simulink model "DC_motor_model"  (R2023a)
settings: Solver=VariableStepAuto  StartTime=0.0  StopTime=10  FixedStep=1/20000  MaxStep=1/10000  RelTol=1e-3
undefined symbols (not defined in the file or in its folder): sigbuilder_block
settings Model: Creator=SC34573  LastModifiedBy=Test
settings SolverCC: ZeroCrossAlgorithm=Adaptive  AlgebraicLoopSolver=TrustRegion
settings DebuggingCC: IgnoredZcDiagnostic=none  UnconnectedInputMsg=warning  UnconnectedOutputMsg=warning  UnconnectedLineMsg=warning
settings ModelReferenceCC: EnableRefExpFcnMdlSchedulingChecks=on
settings RTWCC: DLArmComputeVersion=19.05

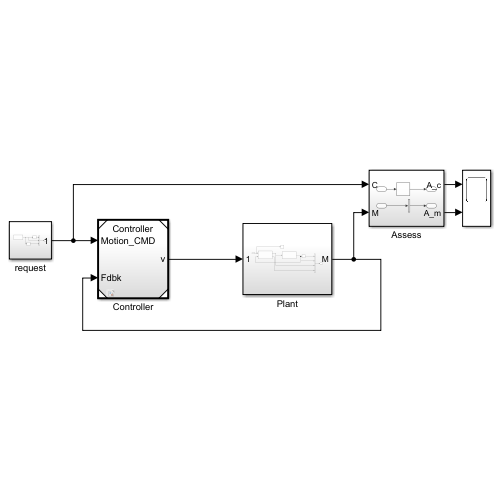
[thumbnail: Simulink's stored preview of the top-level diagram]
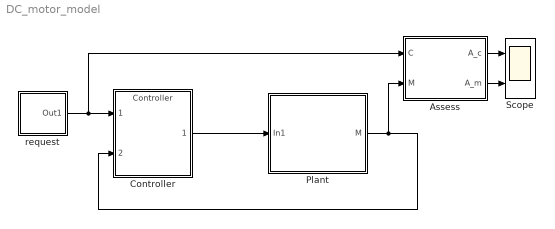
== system DC_motor_model ==
  Assess : Subsystem
  Controller : ModelReference  ModelNameDialog=Controller  SimulationMode=Normal  ModelReferenceVersion=1.31
  Plant : Subsystem
  Scope : Scope  NumInputPorts=2
  request : Subsystem
  wires:
  request/1(Out1) -> Assess/1(C), Controller/1
  Controller/1 -> Plant/1(In1)
  Plant/1(M) -> Controller/2, Assess/2(M)
  Assess/1(A_c) -> Scope/1
  Assess/2(A_m) -> Scope/2

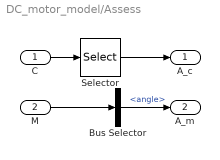
== system DC_motor_model/Assess ==
  C : Inport
  M : Inport  Port=2
  Bus Selector : BusSelector  OutputSignals=angle
  Selector : Selector  InputPortWidth=3  IndexOptions=Index vector (dialog)  Indices=1  OutputSizes=1
  A_c : Outport
  A_m : Outport  Port=2
  wires:
  Selector/1 -> A_c/1
  C/1 -> Selector/1
  M/1 -> Bus Selector/1
  Bus Selector/1 -> A_m/1  "<angle>"

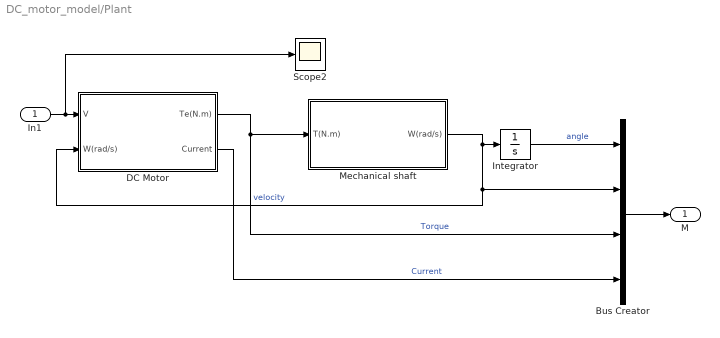
== system DC_motor_model/Plant ==
  In1 : Inport
  Bus Creator : BusCreator  Inputs=4
  "DC Motor " : Subsystem  mask{Vn=30, Tstall=20, wNL=20, L=1e-10}
      mask prompts: Vn "Nominal Voltage"; Tstall "Stall Torque(N.m)"; wNL "No Load Speed(rad/s)"; L "Inductance(H)"
      mask init:
      | K=Vn/wNL;
      | R=Vn^2/wNL/Tstall;
  Integrator : Integrator
  Mechanical shaft : Subsystem  mask{J=1, b=0}
      mask prompts: J "Shaft inertia(Kg.m^2)"; b "Damping Coefficient"
  Scope2 : Scope
  M : Outport
  wires:
  Mechanical shaft/1(W(rad/s)) -> "DC Motor "/2(W(rad/s)), Bus Creator/2, Integrator/1  "velocity"
  In1/1 -> Scope2/1, "DC Motor "/1(V)
  "DC Motor "/1(Te(N.m)) -> Bus Creator/3, Mechanical shaft/1(T(N.m))  "Torque"
  Integrator/1 -> Bus Creator/1  "angle"
  "DC Motor "/2(Current) -> Bus Creator/4  "Current"
  Bus Creator/1 -> M/1

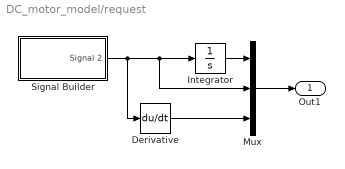
== system DC_motor_model/request ==
  Derivative : Derivative
  Integrator : Integrator
  Mux : Mux  Inputs=3
  Signal Builder : Subsystem  Tag=STV Subsys  LoadFcn=sigbuilder_block('load');  StartFcn=sigbuilder_block('start');  StopFcn=sigbuilder_block('stop');  ClipboardFcn=sigbuilder_block('clipboard');  mask(Sigbuilder block){tuvar=[0:10]}
      mask help: Simulink:masks:SigbuilderBlock_MD
      mask init:
      | if ~strcmp(get_param(bdroot(gcbh),'SimulationStatus'),'stopped') tuvar = sigbuilder_block('maskInit'); end
      settings: CopyFcn=sigbuilder_block('copy');  DeleteFcn=sigbuilder_block('delete');  ModelCloseFcn=sigbuilder_block('modelClose');  PreSaveFcn=sigbuilder_block('preSave');  PauseFcn=sigbuilder_block('pause');  ContinueFcn=sigbuilder_block('continue');  NameChangeFcn=sigbuilder_block('namechange');  OpenFcn=sigbuilder_block('open',[6 22.5 1420.5 635.25 ]);  CloseFcn=sigbuilder_block('close');
      mask Display: plot(0, 0, 100, 100,[2, 2, 32, 32, 2], [68, 8, 8, 68, 68],[32, 2], [38, 38], [32, 19, 2],[53, 60, 44], [32, 17, 17, 2],[16, 16, 31, 31]);txt = getActiveGroup(gcbh);text(2, 100, txt,'verticalAlignment', 'top');
  Out1 : Outport
  wires:
  Signal Builder/1(Signal 2) -> Mux/2, Integrator/1, Derivative/1
  Integrator/1 -> Mux/1
  Derivative/1 -> Mux/3
  Mux/1 -> Out1/1

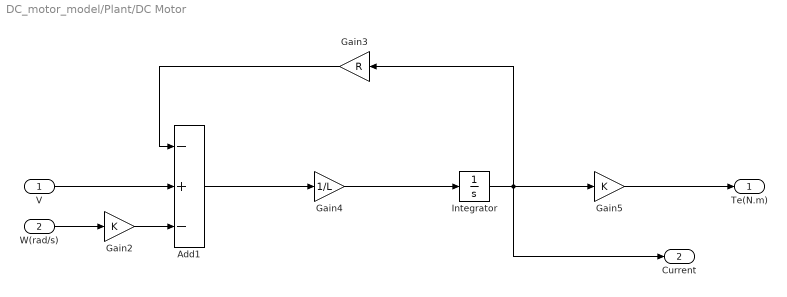
== system DC_motor_model/Plant/DC Motor  ==
  V : Inport
  W(rad/s) : Inport  Port=2
  Add1 : Sum  Inputs=-+-
  Gain2 : Gain  Gain=K
  Gain3 : Gain  Gain=R
  Gain4 : Gain  Gain=1/L
  Gain5 : Gain  Gain=K
  Integrator : Integrator
  Te(N.m) : Outport
  Current : Outport  Port=2
  wires:
  Integrator/1 -> Current/1, Gain5/1, Gain3/1
  V/1 -> Add1/2
  Add1/1 -> Gain4/1
  Gain4/1 -> Integrator/1
  W(rad/s)/1 -> Gain2/1
  Gain5/1 -> Te(N.m)/1
  Gain2/1 -> Add1/3
  Gain3/1 -> Add1/1

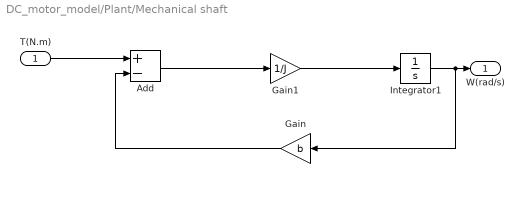
== system DC_motor_model/Plant/Mechanical shaft ==
  T(N.m) : Inport
  Add : Sum  Inputs=+-
  Gain : Gain  Gain=b
  Gain1 : Gain  Gain=1/J
  Integrator1 : Integrator
  W(rad/s) : Outport
  wires:
  Integrator1/1 -> Gain/1, W(rad/s)/1
  Gain/1 -> Add/2
  Add/1 -> Gain1/1
  Gain1/1 -> Integrator1/1
  T(N.m)/1 -> Add/1

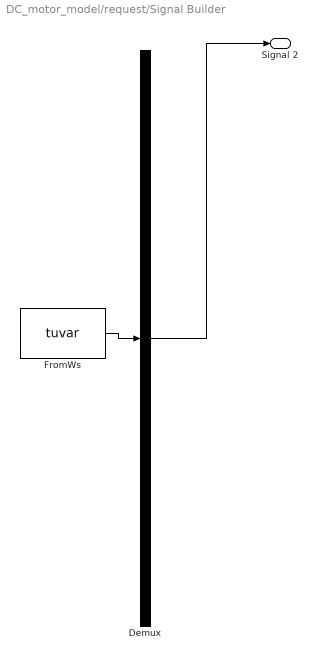
== system DC_motor_model/request/Signal Builder ==
  Demux : Demux  Tag=STV Demux  Outputs=1
      settings: DisplayOption=none
  FromWs : FromWorkspace  Tag=STV FromWs  VariableName=tuvar
      SigBuilderData=|
      | common.afterFinalStr = 'Extrapolate'
      | common.sampleTime = 0
      | dataSet.timeRange = [0 10]
      | dataSet.name = 'Group 1'
      | sbobj.Groups.Name = 'Group 1'
      | sbobj.Groups.Signals.Name = 'Signal 2'
      | sbobj.Groups.Signals.XData = [0 0.02002002002 0.04004004004 0.0600600600601 0.0800800800801 0.1001001001 0.12012012012 0.14014014014 0.16016016016 0.18018018018 0.2002002002 0.22022022022 ... (501 elements, 1x501)]
      | sbobj.Groups.Signals.YData = [0 0.0251577332643 0.050314471355 0.0754692191379 0.100620981558 0.125768763676 0.150911570715 0.17604840809 0.201178281453 0.226300196735 0.251413160178 0.276516178379 ... (501 elements, 1x501)]
  Signal 2 : Outport  Tag=STV Outport
  wires:
  FromWs/1 -> Demux/1
  Demux/1 -> Signal 2/1
